simulink model "WT_DATA_DRIVEN"  (R2025a)
settings: Solver=ode4  StartTime=0.0  StopTime=11  FixedStep=0.1  RelTol=1e-3
settings Model: Creator=hero  LastModifiedBy=hero

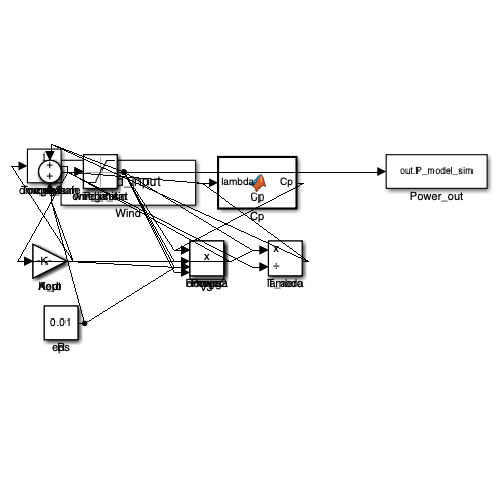
[thumbnail: Simulink's stored preview of the top-level diagram]
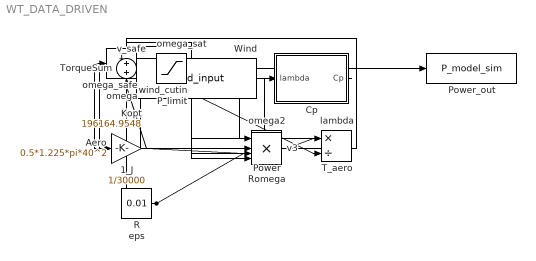
== system WT_DATA_DRIVEN ==
  1_J : Gain  Gain=1/30000
  Aero : Gain  Gain=0.5*1.225*pi*40^2
  Cp : MATLAB Function  TreatAsAtomicUnit=on
  Kopt : Gain  Gain=196164.9548
  P_limit : Saturate  UpperLimit=652.7945  LowerLimit=0
  Power : Product
  Power_out : ToWorkspace  VariableName=P_model_sim  SampleTime=-1
  R : Constant  Value=40
  Romega : Product
  T_aero : Product  Inputs=*/
  TorqueSum : Sum  Inputs=+-
  Wind : FromWorkspace  VariableName=wind_input
  eps : Constant  Value=0.01
  lambda : Product  Inputs=*/
  omega : Integrator  InitialCondition=10
  omega2 : Product
  omega_safe : Sum
  omega_sat : Saturate  UpperLimit=100  LowerLimit=0.1
  v3 : Product  Inputs=3
  v_safe : Sum
  wind_cutin : Saturate  UpperLimit=25  LowerLimit=4.8
  wires:
  Wind/1 -> wind_cutin/1
  wind_cutin/1 -> v3/1, v3/2, v3/3, v_safe/1
  eps/1 -> v_safe/2, omega_safe/2
  omega/1 -> omega_sat/1
  omega_sat/1 -> Romega/1, omega_safe/1, omega2/1, omega2/2
  R/1 -> Romega/2
  Romega/1 -> lambda/1
  v_safe/1 -> lambda/2
  lambda/1 -> Cp/1(lambda)
  Cp/1(Cp) -> Power/1
  v3/1 -> Aero/1
  Aero/1 -> Power/2
  Power/1 -> P_limit/1
  P_limit/1 -> Power_out/1, T_aero/1
  omega_safe/1 -> T_aero/2
  T_aero/1 -> TorqueSum/1
  omega2/1 -> Kopt/1
  Kopt/1 -> TorqueSum/2
  TorqueSum/1 -> 1_J/1
  1_J/1 -> omega/1

== matlab function WT_DATA_DRIVEN/Cp ==
  data: lambda input; Cp output
function Cp = Cp(lambda)
lambda = max(lambda,0.1);
lambda = min(lambda,12);
p = [-21998.5640971324,731324.3761698254,-9570129.3243424594,61312289.9676896632,-190810752.9494479895,227742849.0204843581];
Cp = polyval(p,lambda);
Cp = max(min(Cp,0.6),0);
end
